simulink model "CAN_Model_v8"  (R2018b)
settings: Solver=VariableStepAuto  StartTime=0.0  StopTime=SimTime  RelTol=1e-3
values from neighbouring files (symbols this model uses):
  ID = [1,1,1,1,1,0,0,1,1,1,1]    [CAN_ModelMat.m]    (also in CAN_ModelMatv2.m; stuff.m = [ID(1:i) 0 ID(i+1:end)])
  ID_Rx = [1,1,1,1,0,0,1,1,1,1,1]    [CAN_ModelMat.m]    (also in CAN_ModelMatv2.m)
  NodesID = [ 0,0,1,1,0,1,1,0,0,1,1 ... (first row only)    [CAN_ModelMat.m]    (also in CAN_ModelMatv2.m)
  RTS_Inc = round(SimTime / CLK / NumOfFrames)    [CAN_ModelMat.m]    (also in CAN_ModelMatv2.m)
  time = NodeTiming / CLK    (= 5000)    [CAN_ModelMat.m]    (also in CAN_ModelMatv2.m)
libraries: simulink_extras x1
(part 1 of 2)
settings Model: Creator=Emiliano  LastModifiedBy=MAX_1

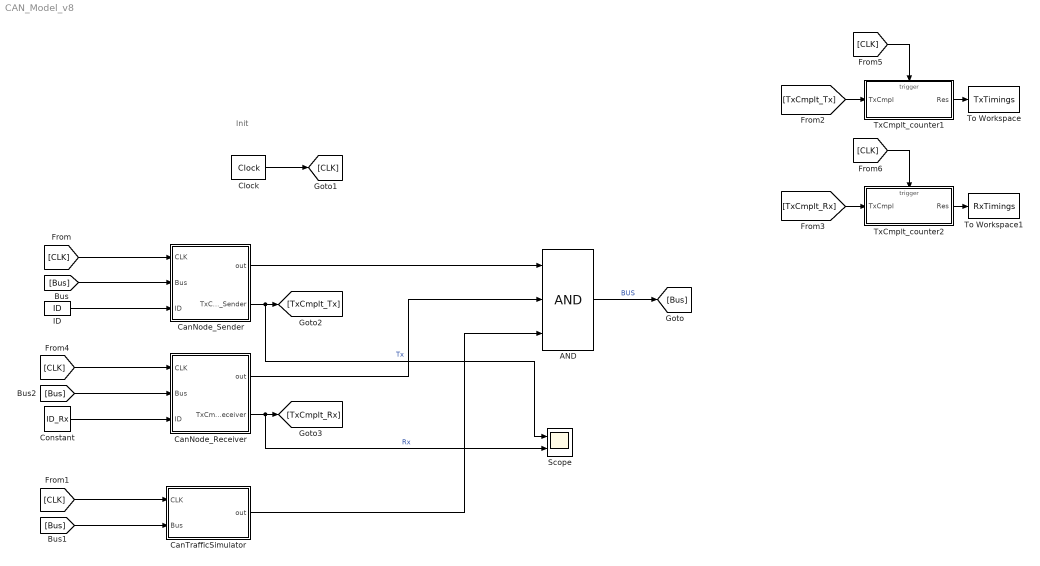
== system CAN_Model_v8 ==
  note: Init
  AND : Logic  Inputs=3  IconShape=distinctive  AllPortsSameDT=off  OutDataTypeStr=boolean
  CanNode_Receiver : Subsystem
  CanNode_Sender : Subsystem
  CanTrafficSimulator : Subsystem
  Clock : simulink_extras/Flip Flops/Clock  period=CLK
  Constant : Constant  Value=ID_Rx
  ID : Constant  Value=ID
  Scope : Scope  NumInputPorts=2
  To Workspace : ToWorkspace  VariableName=TxTimings  SaveFormat=Timeseries  SampleTime=-1
  To Workspace1 : ToWorkspace  VariableName=RxTimings  SaveFormat=Timeseries  SampleTime=-1
  TxCmplt_counter1 : Subsystem  TreatAsAtomicUnit=on
  TxCmplt_counter2 : Subsystem  TreatAsAtomicUnit=on
  wires:
  AND/1 -> [Bus]  "BUS"
  Clock/1 -> [CLK]
  [CLK] -> CanNode_Sender/1(CLK)
  [Bus] -> CanNode_Sender/2(Bus)
  ID/1 -> CanNode_Sender/3(ID)
  CanNode_Sender/1(out) -> AND/1
  [CLK] -> CanNode_Receiver/1(CLK)
  [Bus] -> CanNode_Receiver/2(Bus)
  Constant/1 -> CanNode_Receiver/3(ID)
  CanNode_Receiver/1(out) -> AND/2
  [CLK] -> CanTrafficSimulator/1(CLK)
  [Bus] -> CanTrafficSimulator/2("Bus ")
  CanTrafficSimulator/1(out) -> AND/3
  CanNode_Sender/2(TxCmplt_Sender) -> Scope/1, [TxCmplt_Tx]  "Tx"
  [CLK] -> TxCmplt_counter1/Trigger
  [CLK] -> TxCmplt_counter2/Trigger
  [TxCmplt_Rx] -> TxCmplt_counter2/1(TxCmpl)
  [TxCmplt_Tx] -> TxCmplt_counter1/1(TxCmpl)
  TxCmplt_counter1/1(Res) -> To Workspace/1
  TxCmplt_counter2/1(Res) -> To Workspace1/1
  CanNode_Receiver/2(TxCmplt_Receiver) -> Scope/2, [TxCmplt_Rx]  "Rx"

== system CAN_Model_v8/CanNode_Receiver ==
  CLK : Inport
  Bus : Inport  Port=2
  ID : Inport  Port=3
  CanNode : Subsystem
  Payload 1 : Constant  Value=[0,0,0,1,0,0,0,1,1,1,0,0,0,1,1,0,1,0,0,1,0,0,1,1,0,0,0,1,0,1,0,1,0,0,0,0,1,0,0,1,0,1,0,1,1,0,0,0,0,1,0,0,0,1,1,0,1,0,0,1,0,0,0,1]
  RTR2 : Constant
  Scope : Scope
  Triggered Subsystem2 : Subsystem  TreatAsAtomicUnit=on
  out : Outport
  TxCmplt_Receiver : Outport  Port=2
  wires:
  CanNode/3(txCmplt) -> TxCmplt_Receiver/1, Triggered Subsystem2/2(TxCmplt)  "TxCmplt_Receiver"
  Payload 1/1 -> CanNode/5(Data)
  RTR2/1 -> CanNode/4(RTR)
  CLK/1 -> Triggered Subsystem2/Trigger, CanNode/1(CLK)
  CanNode/2(DeStuffedFrame) -> Triggered Subsystem2/1(RxFrame)
  Triggered Subsystem2/1(RTS) -> Scope/1, CanNode/6("ReadyToSend ")  "RTS"
  CanNode/4(EOF) -> Triggered Subsystem2/3(EOF)
  ID/1 -> CanNode/3(ID)
  CanNode/1("TxBus ") -> out/1  "out"
  Bus/1 -> CanNode/2(Bus)

== system CAN_Model_v8/CanNode_Sender ==
  CLK : Inport
  Bus : Inport  Port=2
  ID : Inport  Port=3
  CanNode : Subsystem
  "Payload " : Constant  Value=[0,0,0,1,0,0,0,1,1,1,0,0,0,1,1,0,1,0,0,1,0,0,1,1,0,0,0,1,0,1,0,1,0,0,0,0,1,0,0,1,0,1,0,1,1,0,0,0,0,1,0,0,0,1,1,0,1,0,0,1,0,0,0,1]
  RTR : Constant
  RTS_Manager : Subsystem  TreatAsAtomicUnit=on
  Terminator : Terminator
  out : Outport
  TxCmplt_Sender : Outport  Port=2
  wires:
  Bus/1 -> CanNode/2(Bus)
  CLK/1 -> CanNode/1(CLK), RTS_Manager/Trigger
  "Payload "/1 -> CanNode/5(Data)
  CanNode/2(DeStuffedFrame) -> Terminator/1
  CanNode/1("TxBus ") -> out/1  "out"
  ID/1 -> CanNode/3(ID)
  CanNode/3(txCmplt) -> TxCmplt_Sender/1, RTS_Manager/1(TxCmplt)  "TxCmplt_Sender"
  RTS_Manager/1(RTS) -> CanNode/6("ReadyToSend ")  "RTS"
  RTR/1 -> CanNode/4(RTR)

== system CAN_Model_v8/CanTrafficSimulator ==
  CLK : Inport
  "Bus " : Inport  Port=2
  CanNode : Subsystem
  Payload 1 : Constant  Value=[0,0,0,1,0,0,0,1,1,1,0,0,0,1,1,0,1,0,0,1,0,0,1,1,0,0,0,1,0,1,0,1,0,0,0,0,1,0,0,1,0,1,0,1,1,0,0,0,0,1,0,0,0,1,1,0,1,0,0,1,0,0,0,1]
  RTR1 : Constant
  Terminator : Terminator
  To Workspace : ToWorkspace  VariableName=DeStuffed  SaveFormat=Timeseries  SampleTime=-1
  Triggered Subsystem : Subsystem  TreatAsAtomicUnit=on
  out : Outport
  wires:
  RTR1/1 -> CanNode/4(RTR)
  CanNode/2(DeStuffedFrame) -> To Workspace/1
  Triggered Subsystem/1(ID) -> CanNode/3(ID)
  CanNode/1("TxBus ") -> out/1  "out"
  CLK/1 -> CanNode/1(CLK), Triggered Subsystem/Trigger
  CanNode/3(txCmplt) -> Triggered Subsystem/1(TxCmplt)  "TxCmplt"
  "Bus "/1 -> CanNode/2(Bus)
  Triggered Subsystem/3(RTS) -> CanNode/6("ReadyToSend ")  "RTS_Traffic"
  Payload 1/1 -> CanNode/5(Data)
  Triggered Subsystem/2(RandPayload) -> Terminator/1

== system CAN_Model_v8/TxCmplt_counter1 ==
  TxCmpl : Inport
  Trigger : TriggerPort  VariantControl=Variant
  MATLAB Function : MATLAB Function  TreatAsAtomicUnit=on
  Memory : Memory  InitialCondition=1  InheritSampleTime=on
  Memory1 : Memory  InheritSampleTime=on
  Memory2 : Memory  InitialCondition=[0,0,0,0,0,0,0,0,0,0,0,0,0,0,0,0,0,0,0,0]  InheritSampleTime=on
  Res : Outport
  wires:
  MATLAB Function/3(nextIndex) -> Memory/1
  MATLAB Function/2(nextCount) -> Memory1/1
  MATLAB Function/1(nextRes) -> Res/1, Memory2/1
  Memory/1 -> MATLAB Function/4(index)
  Memory1/1 -> MATLAB Function/3(count)
  Memory2/1 -> MATLAB Function/2(Res)
  TxCmpl/1 -> MATLAB Function/1(TxCmplt)

== system CAN_Model_v8/TxCmplt_counter2 ==
  TxCmpl : Inport
  Trigger : TriggerPort  VariantControl=Variant
  MATLAB Function : MATLAB Function  TreatAsAtomicUnit=on
  Memory : Memory  InitialCondition=1  InheritSampleTime=on
  Memory1 : Memory  InheritSampleTime=on
  Memory2 : Memory  InitialCondition=[0,0,0,0,0,0,0,0,0,0,0,0,0,0,0,0,0,0,0,0]  InheritSampleTime=on
  Res : Outport
  wires:
  MATLAB Function/3(nextIndex) -> Memory/1
  MATLAB Function/2(nextCount) -> Memory1/1
  MATLAB Function/1(nextRes) -> Res/1, Memory2/1
  Memory/1 -> MATLAB Function/4(index)
  Memory1/1 -> MATLAB Function/3(count)
  Memory2/1 -> MATLAB Function/2(Res)
  TxCmpl/1 -> MATLAB Function/1(TxCmplt)

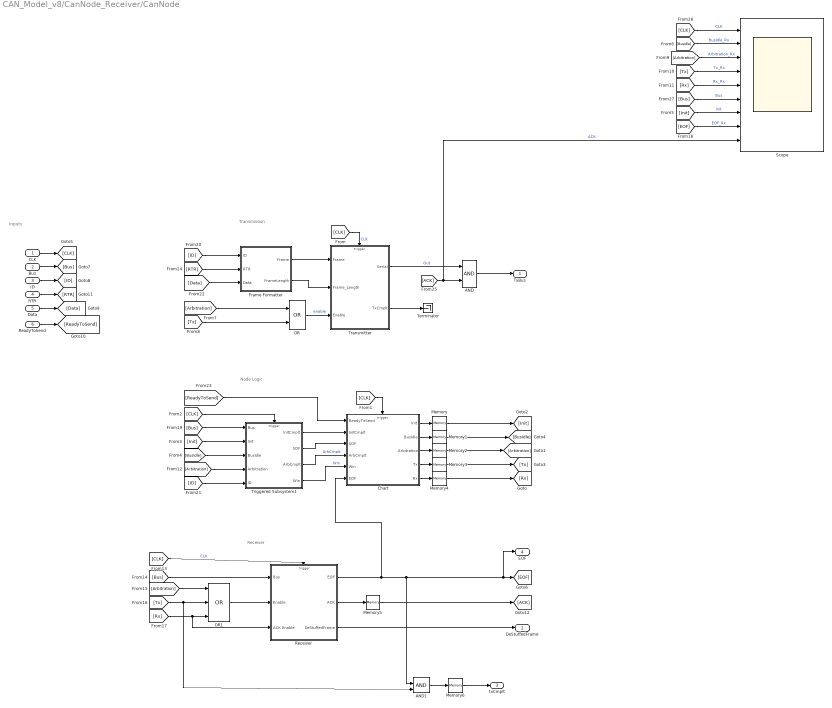
== system CAN_Model_v8/CanNode_Receiver/CanNode ==
  note: Transmission
  note: Node Logic
  note: Receiver
  note: Inputs
  CLK : Inport
  Bus : Inport  Port=2
  ID : Inport  Port=3
  RTR : Inport  Port=4
  Data : Inport  Port=5
  "ReadyToSend " : Inport  Port=6
  AND : Logic  IconShape=distinctive  AllPortsSameDT=off  OutDataTypeStr=boolean
  AND1 : Logic  IconShape=distinctive  AllPortsSameDT=off  OutDataTypeStr=boolean
  Chart : Stateflow chart  TreatAsAtomicUnit=on
  Frame Formatter : Subsystem
  Memory{,1..5} (6 alike) : Memory
  Memory6 : Memory  InheritSampleTime=on
  OR : Logic  Operator=OR  IconShape=distinctive  AllPortsSameDT=off  OutDataTypeStr=boolean
  OR1 : Logic  Operator=OR  Inputs=3  IconShape=distinctive  AllPortsSameDT=off  OutDataTypeStr=boolean
  Receiver : Subsystem  TreatAsAtomicUnit=on
  Scope : Scope  NumInputPorts=9
  Terminator : Terminator
  Transmitter : Subsystem  TreatAsAtomicUnit=on
  Triggered Subsystem1 : Subsystem  TreatAsAtomicUnit=on
  "TxBus " : Outport
  DeStuffedFrame : Outport  Port=2
  txCmplt : Outport  Port=3
  EOF : Outport  Port=4
  wires:
  [CLK] -> Chart/Trigger
  [Arbitration] -> OR/1
  [Tx] -> OR/2
  OR/1 -> Transmitter/3(Enable)  "enable"
  Chart/5(" Rx") -> Memory4/1
  Chart/3(" Arbitration") -> Memory2/1
  Chart/1(" Init") -> Memory/1
  Chart/4(" Tx") -> Memory3/1
  Chart/2(" BusIdle") -> Memory1/1
  CLK/1 -> [CLK]
  [CLK] -> Transmitter/Trigger  "CLK"
  [CLK] -> Triggered Subsystem1/Trigger
  [Init] -> Triggered Subsystem1/2(Init)
  [BusIdle] -> Triggered Subsystem1/3(BusIdle)
  Triggered Subsystem1/2(SOF) -> Chart/3(SOF)
  Triggered Subsystem1/3("ArbCmplt ") -> Chart/4(ArbCmplt)  "ArbCmplt"
  [CLK] -> Scope/1  "CLK"
  [BusIdle] -> Scope/2  "BusIdle_Rx"
  [Arbitration] -> Scope/3  "Arbitration_Rx"
  [Tx] -> Scope/4  "Tx_Rx"
  [Rx] -> Scope/5  "Rx_Rx"
  Memory/1 -> [Init]
  Memory1/1 -> [BusIdle]
  Memory2/1 -> [Arbitration]
  Memory3/1 -> [Tx]
  Memory4/1 -> [Rx]
  Transmitter/1(Serial) -> AND/1  "Out"
  [Arbitration] -> Triggered Subsystem1/4(Arbitration)
  [CLK] -> Receiver/Trigger  "CLK"
  [Bus] -> Receiver/1(Bus)
  [Arbitration] -> OR1/1
  [Tx] -> AND1/2, OR1/2
  Receiver/1(EOF) -> Chart/6(EOF), AND1/1, EOF/1, [EOF]
  [EOF] -> Scope/8  "EOF_Rx"
  Bus/1 -> [Bus]
  [Bus] -> Triggered Subsystem1/1(Bus)
  Frame Formatter/1(Frame) -> Transmitter/1("Frame ")
  Frame Formatter/2("FrameLength ") -> Transmitter/2(Frame_Length)
  ID/1 -> [ID]
  [ID] -> Frame Formatter/1(ID)
  [ID] -> Triggered Subsystem1/5(ID)
  Data/1 -> [Data]
  "ReadyToSend "/1 -> [ReadyToSend]
  [ReadyToSend] -> Chart/1(ReadyToSend)
  [Data] -> Frame Formatter/3(Data)
  RTR/1 -> [RTR]
  [RTR] -> Frame Formatter/2(RTR)
  Receiver/2(ACK) -> Memory5/1
  Triggered Subsystem1/4(Win) -> Chart/5(Win)  "Win"
  Memory5/1 -> [ACK]
  AND/1 -> "TxBus "/1
  [ACK] -> Scope/9, AND/2  "ACK"
  Triggered Subsystem1/1(InitCmplt) -> Chart/2(InitCmplt)
  [Init] -> Scope/7  "Init"
  Receiver/3(DeStuffedFrame) -> DeStuffedFrame/1
  OR1/1 -> Receiver/2(Enable)
  [Rx] -> Receiver/3(ACK Enable), OR1/3
  Transmitter/2(TxCmplt) -> Terminator/1
  AND1/1 -> Memory6/1
  Memory6/1 -> txCmplt/1
  [Bus] -> Scope/6  "Bus"

== system CAN_Model_v8/CanNode_Receiver/Triggered Subsystem2 ==
  RxFrame : Inport
  TxCmplt : Inport  Port=2
  EOF : Inport  Port=3
  Trigger : TriggerPort  VariantControl=Variant
  Constant : Constant  Value=ID
  MATLAB Function : MATLAB Function  TreatAsAtomicUnit=on
  Memory1 : Memory  InheritSampleTime=on
  Scope : Scope
  RTS : Outport
  wires:
  MATLAB Function/1(nextRTS) -> Memory1/1, RTS/1
  TxCmplt/1 -> MATLAB Function/2(TxCmplt)
  Memory1/1 -> MATLAB Function/5(RTS)
  EOF/1 -> MATLAB Function/3(EOF)
  RxFrame/1 -> MATLAB Function/4(RxFrame)
  Constant/1 -> MATLAB Function/1(MasterID)
  MATLAB Function/2(out) -> Scope/1

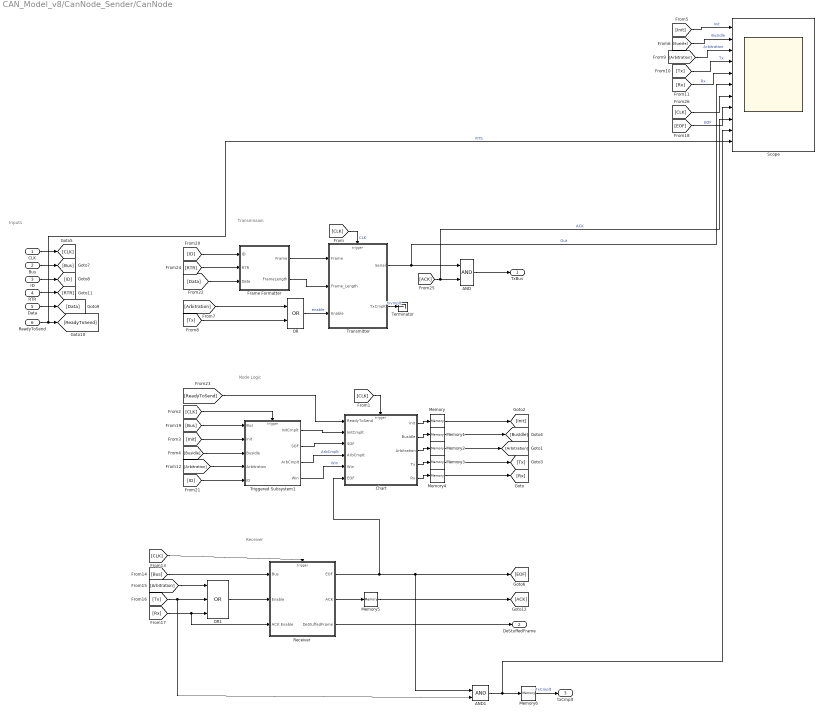
== system CAN_Model_v8/CanNode_Sender/CanNode ==
  note: Transmission
  note: Node Logic
  note: Receiver
  note: Inputs
  CLK : Inport
  Bus : Inport  Port=2
  ID : Inport  Port=3
  RTR : Inport  Port=4
  Data : Inport  Port=5
  "ReadyToSend " : Inport  Port=6
  AND : Logic  IconShape=distinctive  AllPortsSameDT=off  OutDataTypeStr=boolean
  AND1 : Logic  IconShape=distinctive  AllPortsSameDT=off  OutDataTypeStr=boolean
  Chart : Stateflow chart  TreatAsAtomicUnit=on
  Frame Formatter : Subsystem
  Memory{,1..5} (6 alike) : Memory
  Memory6 : Memory  InheritSampleTime=on
  OR : Logic  Operator=OR  IconShape=distinctive  AllPortsSameDT=off  OutDataTypeStr=boolean
  OR1 : Logic  Operator=OR  Inputs=3  IconShape=distinctive  AllPortsSameDT=off  OutDataTypeStr=boolean
  Receiver : Subsystem  TreatAsAtomicUnit=on
  Scope : Scope  NumInputPorts=11
  Terminator : Terminator
  Transmitter : Subsystem  TreatAsAtomicUnit=on
  Triggered Subsystem1 : Subsystem  TreatAsAtomicUnit=on
  "TxBus " : Outport
  DeStuffedFrame : Outport  Port=2
  txCmplt : Outport  Port=3
  wires:
  [CLK] -> Chart/Trigger
  [Arbitration] -> OR/1
  [Tx] -> OR/2
  OR/1 -> Transmitter/3(Enable)  "enable"
  Chart/5(" Rx") -> Memory4/1
  Chart/3(" Arbitration") -> Memory2/1
  Chart/1(" Init") -> Memory/1
  Chart/4(" Tx") -> Memory3/1
  Chart/2(" BusIdle") -> Memory1/1
  CLK/1 -> [CLK]
  [CLK] -> Transmitter/Trigger  "CLK"
  [CLK] -> Triggered Subsystem1/Trigger
  [Init] -> Triggered Subsystem1/2(Init)
  [BusIdle] -> Triggered Subsystem1/3(BusIdle)
  Triggered Subsystem1/2(SOF) -> Chart/3(SOF)
  Triggered Subsystem1/3("ArbCmplt ") -> Chart/4(ArbCmplt)  "ArbCmplt"
  [Init] -> Scope/1  "Init"
  [BusIdle] -> Scope/2  "BusIdle"
  [Arbitration] -> Scope/3  "Arbitration"
  [Tx] -> Scope/4  "Tx"
  [Rx] -> Scope/5  "Rx"
  Memory/1 -> [Init]
  Memory1/1 -> [BusIdle]
  Memory2/1 -> [Arbitration]
  Memory3/1 -> [Tx]
  Memory4/1 -> [Rx]
  Transmitter/1(Serial) -> Scope/6, AND/1  "Out"
  [Arbitration] -> Triggered Subsystem1/4(Arbitration)
  [CLK] -> Receiver/Trigger
  [Bus] -> Receiver/1(Bus)
  [Arbitration] -> OR1/1
  [Tx] -> AND1/2, OR1/2
  Receiver/1(EOF) -> Chart/6(EOF), AND1/1, [EOF]
  [EOF] -> Scope/8  "EOF"
  Bus/1 -> [Bus]
  [Bus] -> Triggered Subsystem1/1(Bus)
  Frame Formatter/1(Frame) -> Transmitter/1("Frame ")
  Frame Formatter/2("FrameLength ") -> Transmitter/2(Frame_Length)
  ID/1 -> [ID]
  [ID] -> Frame Formatter/1(ID)
  [ID] -> Triggered Subsystem1/5(ID)
  Data/1 -> [Data]
  "ReadyToSend "/1 -> Scope/11, [ReadyToSend]  "RTS"
  [ReadyToSend] -> Chart/1(ReadyToSend)
  [Data] -> Frame Formatter/3(Data)
  RTR/1 -> [RTR]
  [RTR] -> Frame Formatter/2(RTR)
  Receiver/2(ACK) -> Memory5/1
  Triggered Subsystem1/4(Win) -> Chart/5(Win)  "Win"
  Memory5/1 -> [ACK]
  AND/1 -> "TxBus "/1
  [ACK] -> Scope/9, AND/2  "ACK"
  Triggered Subsystem1/1(InitCmplt) -> Chart/2(InitCmplt)
  [CLK] -> Scope/7
  Receiver/3(DeStuffedFrame) -> DeStuffedFrame/1
  OR1/1 -> Receiver/2(Enable)
  [Rx] -> Receiver/3(ACK Enable), OR1/3
  Transmitter/2(TxCmplt) -> Terminator/1  "txvmplt"
  AND1/1 -> Scope/10, Memory6/1
  Memory6/1 -> txCmplt/1  "TxCmplt"

== system CAN_Model_v8/CanNode_Sender/RTS_Manager ==
  TxCmplt : Inport
  Trigger : TriggerPort  VariantControl=Variant
  Constant : Constant  Value=time
  MATLAB Function : MATLAB Function  TreatAsAtomicUnit=on
  Memory : Memory  InheritSampleTime=on
  Memory1 : Memory  InheritSampleTime=on
  Memory2 : Memory  InheritSampleTime=on
  RTS : Outport
  wires:
  MATLAB Function/1(nextRTS) -> Memory1/1, RTS/1
  Constant/1 -> MATLAB Function/1(Timer)
  TxCmplt/1 -> MATLAB Function/2(TxCmplt)
  MATLAB Function/2(nextCount) -> Memory/1
  Memory/1 -> MATLAB Function/4(Count)
  Memory1/1 -> MATLAB Function/3(RTS)
  MATLAB Function/3(nextNumPackets) -> Memory2/1
  Memory2/1 -> MATLAB Function/5(numPackets)

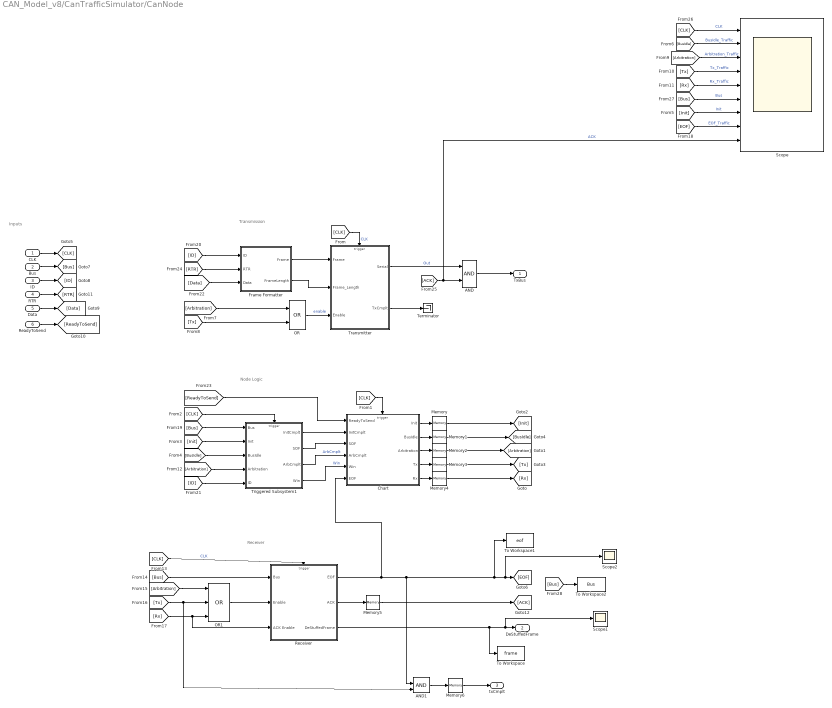
== system CAN_Model_v8/CanTrafficSimulator/CanNode ==
  note: Transmission
  note: Node Logic
  note: Receiver
  note: Inputs
  CLK : Inport
  Bus : Inport  Port=2
  ID : Inport  Port=3
  RTR : Inport  Port=4
  Data : Inport  Port=5
  "ReadyToSend " : Inport  Port=6
  AND : Logic  IconShape=distinctive  AllPortsSameDT=off  OutDataTypeStr=boolean
  AND1 : Logic  IconShape=distinctive  AllPortsSameDT=off  OutDataTypeStr=boolean
  Chart : Stateflow chart  TreatAsAtomicUnit=on
  Frame Formatter : Subsystem
  Memory{,1..5} (6 alike) : Memory
  Memory6 : Memory  InheritSampleTime=on
  OR : Logic  Operator=OR  IconShape=distinctive  AllPortsSameDT=off  OutDataTypeStr=boolean
  OR1 : Logic  Operator=OR  Inputs=3  IconShape=distinctive  AllPortsSameDT=off  OutDataTypeStr=boolean
  Receiver : Subsystem  TreatAsAtomicUnit=on
  Scope : Scope  NumInputPorts=9
  Scope1 : Scope
  Scope2 : Scope
  Terminator : Terminator
  To Workspace : ToWorkspace  VariableName=frame  SaveFormat=Timeseries  SampleTime=-1
  To Workspace1 : ToWorkspace  VariableName=eof  SaveFormat=Timeseries  SampleTime=-1
  To Workspace2 : ToWorkspace  VariableName=Bus  SaveFormat=Timeseries  SampleTime=-1
  Transmitter : Subsystem  TreatAsAtomicUnit=on
  Triggered Subsystem1 : Subsystem  TreatAsAtomicUnit=on
  "TxBus " : Outport
  DeStuffedFrame : Outport  Port=2
  txCmplt : Outport  Port=3
  wires:
  [CLK] -> Chart/Trigger
  [Arbitration] -> OR/1
  [Tx] -> OR/2
  OR/1 -> Transmitter/3(Enable)  "enable"
  Chart/5(" Rx") -> Memory4/1
  Chart/3(" Arbitration") -> Memory2/1
  Chart/1(" Init") -> Memory/1
  Chart/4(" Tx") -> Memory3/1
  Chart/2(" BusIdle") -> Memory1/1
  CLK/1 -> [CLK]
  [CLK] -> Transmitter/Trigger  "CLK"
  [CLK] -> Triggered Subsystem1/Trigger
  [Init] -> Triggered Subsystem1/2(Init)
  [BusIdle] -> Triggered Subsystem1/3(BusIdle)
  Triggered Subsystem1/2(SOF) -> Chart/3(SOF)
  Triggered Subsystem1/3("ArbCmplt ") -> Chart/4(ArbCmplt)  "ArbCmplt"
  [CLK] -> Scope/1  "CLK"
  [BusIdle] -> Scope/2  "BusIdle_Traffic"
  [Arbitration] -> Scope/3  "Arbitration_Traffic"
  [Tx] -> Scope/4  "Tx_Traffic"
  [Rx] -> Scope/5  "Rx_Traffic"
  Memory/1 -> [Init]
  Memory1/1 -> [BusIdle]
  Memory2/1 -> [Arbitration]
  Memory3/1 -> [Tx]
  Memory4/1 -> [Rx]
  Transmitter/1(Serial) -> AND/1  "Out"
  [Arbitration] -> Triggered Subsystem1/4(Arbitration)
  [CLK] -> Receiver/Trigger  "CLK"
  [Bus] -> Receiver/1(Bus)
  [Arbitration] -> OR1/1
  [Tx] -> AND1/2, OR1/2
  Receiver/1(EOF) -> Chart/6(EOF), AND1/1, To Workspace1/1, Scope2/1, [EOF]
  [EOF] -> Scope/8  "EOF_Traffic"
  Bus/1 -> [Bus]
  [Bus] -> Triggered Subsystem1/1(Bus)
  Frame Formatter/1(Frame) -> Transmitter/1("Frame ")
  Frame Formatter/2("FrameLength ") -> Transmitter/2(Frame_Length)
  ID/1 -> [ID]
  [ID] -> Frame Formatter/1(ID)
  [ID] -> Triggered Subsystem1/5(ID)
  Data/1 -> [Data]
  "ReadyToSend "/1 -> [ReadyToSend]
  [ReadyToSend] -> Chart/1(ReadyToSend)
  [Data] -> Frame Formatter/3(Data)
  RTR/1 -> [RTR]
  [RTR] -> Frame Formatter/2(RTR)
  Receiver/2(ACK) -> Memory5/1
  Triggered Subsystem1/4(Win) -> Chart/5(Win)  "Win"
  Memory5/1 -> [ACK]
  AND/1 -> "TxBus "/1
  [ACK] -> Scope/9, AND/2  "ACK"
  Triggered Subsystem1/1(InitCmplt) -> Chart/2(InitCmplt)
  [Init] -> Scope/7  "Init"
  Receiver/3(DeStuffedFrame) -> To Workspace/1, Scope1/1, DeStuffedFrame/1
  OR1/1 -> Receiver/2(Enable)
  [Rx] -> Receiver/3(ACK Enable), OR1/3
  Transmitter/2(TxCmplt) -> Terminator/1
  AND1/1 -> Memory6/1
  Memory6/1 -> txCmplt/1
  [Bus] -> Scope/6  "Bus"
  [Bus] -> To Workspace2/1

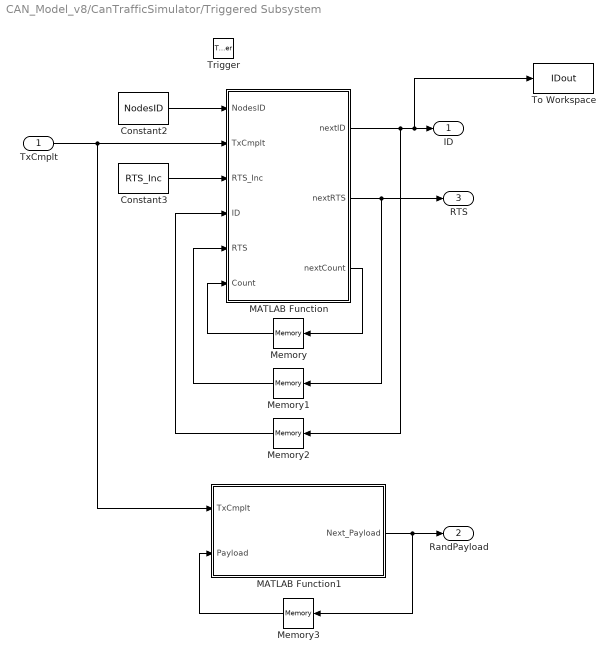
== system CAN_Model_v8/CanTrafficSimulator/Triggered Subsystem ==
  TxCmplt : Inport
  Trigger : TriggerPort  VariantControl=Variant
  Constant2 : Constant  Value=NodesID
  Constant3 : Constant  Value=RTS_Inc
  MATLAB Function : MATLAB Function  TreatAsAtomicUnit=on
  MATLAB Function1 : MATLAB Function  TreatAsAtomicUnit=on
  Memory : Memory  InheritSampleTime=on
  Memory1 : Memory  InheritSampleTime=on
  Memory2 : Memory  InitialCondition=NodesID(1,:)  InheritSampleTime=on
  Memory3 : Memory  InitialCondition=randi([0,1],64, 1)  InheritSampleTime=on
  To Workspace : ToWorkspace  VariableName=IDout  SaveFormat=Timeseries  SampleTime=-1
  ID : Outport
  RandPayload : Outport  Port=2
  RTS : Outport  Port=3
  wires:
  Constant2/1 -> MATLAB Function/1(NodesID)
  MATLAB Function/3(nextCount) -> Memory/1
  Memory/1 -> MATLAB Function/6(Count)
  MATLAB Function/2(nextRTS) -> Memory1/1, RTS/1
  Memory1/1 -> MATLAB Function/5(RTS)
  MATLAB Function/1(nextID) -> To Workspace/1, ID/1, Memory2/1
  Memory2/1 -> MATLAB Function/4(ID)
  Constant3/1 -> MATLAB Function/3(RTS_Inc)
  TxCmplt/1 -> MATLAB Function1/1(TxCmplt), MATLAB Function/2(TxCmplt)
  MATLAB Function1/1(Next_Payload) -> RandPayload/1, Memory3/1
  Memory3/1 -> MATLAB Function1/2(Payload)

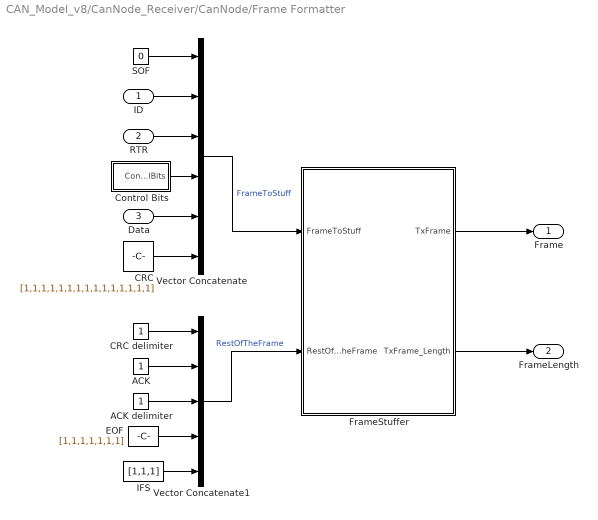
== system CAN_Model_v8/CanNode_Receiver/CanNode/Frame Formatter ==
  ID : Inport
  RTR : Inport  Port=2
  Data : Inport  Port=3
  ACK : Constant
  ACK delimiter : Constant
  CRC : Constant  Value=[1,1,1,1,1,1,1,1,1,1,1,1,1,1,1]
  CRC delimiter : Constant  VectorParams1D=off
  Control Bits : Subsystem
  EOF : Constant  Value=[1,1,1,1,1,1,1]
  FrameStuffer : Subsystem
  IFS : Constant  Value=[1,1,1]
  SOF : Constant  Value=0
  Vector Concatenate : Concatenate  NumInputs=6
  Vector Concatenate1 : Concatenate  NumInputs=5
  Frame : Outport
  "FrameLength " : Outport  Port=2
  wires:
  ID/1 -> Vector Concatenate/2
  RTR/1 -> Vector Concatenate/3
  Vector Concatenate/1 -> FrameStuffer/1(FrameToStuff)  "FrameToStuff"
  FrameStuffer/1(TxFrame) -> Frame/1
  FrameStuffer/2(TxFrame_Length) -> "FrameLength "/1
  SOF/1 -> Vector Concatenate/1
  Control Bits/1(ControlBits) -> Vector Concatenate/4
  Data/1 -> Vector Concatenate/5
  CRC/1 -> Vector Concatenate/6
  CRC delimiter/1 -> Vector Concatenate1/1
  ACK/1 -> Vector Concatenate1/2
  ACK delimiter/1 -> Vector Concatenate1/3
  EOF/1 -> Vector Concatenate1/4
  IFS/1 -> Vector Concatenate1/5
  Vector Concatenate1/1 -> FrameStuffer/2(RestOfTheFrame)  "RestOfTheFrame"

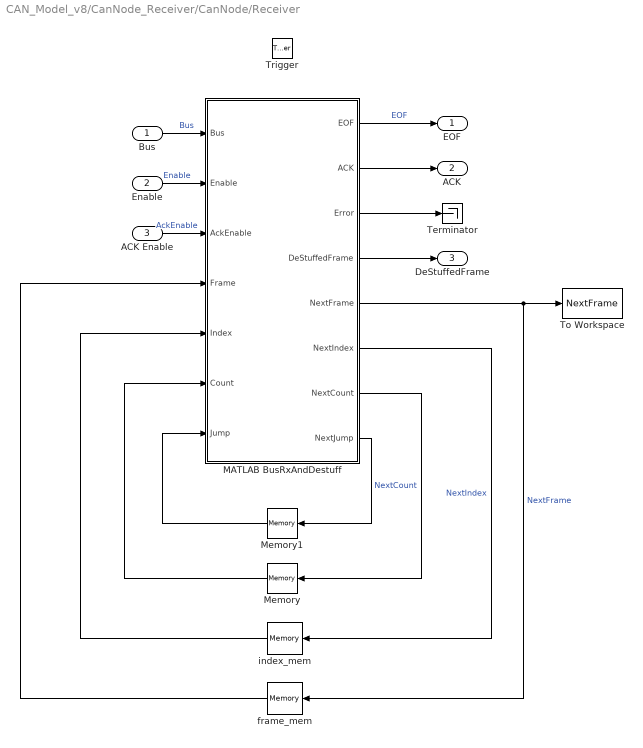
== system CAN_Model_v8/CanNode_Receiver/CanNode/Receiver ==
  Bus : Inport
  Enable : Inport  Port=2
  ACK Enable : Inport  Port=3
  Trigger : TriggerPort  VariantControl=Variant
  MATLAB BusRxAndDestuff : MATLAB Function  TreatAsAtomicUnit=on
  Memory : Memory  InheritSampleTime=on
  Memory1 : Memory  InheritSampleTime=on
  Terminator : Terminator
  To Workspace : ToWorkspace  VariableName=NextFrame  SaveFormat=Timeseries  SampleTime=-1
  frame_mem : Memory  InitialCondition=[0,0,0,0,0,0,0,0,0,0,0,0,0,0,0,0,0,0,0,0,0,0,0,0,0,0,0,0,0,0,0,0,0,0,0,0,0,0,0,0,0,0,0,0,0,0,0,0,0,0,0,0,0,0,0,0,0,0,0,0,0,0,0,0,0,0,0,0,0,0,0,0,0,0,0,0,0,0,0,0,0,0,0,0,0,0,0,0,0,0,0,0,0,0,0,0,0,0,0,0,0,0,0,0,0,0,0,0,0,0,0]  InheritSampleTime=on
  index_mem : Memory  InitialCondition=2  InheritSampleTime=on
  EOF : Outport
  ACK : Outport  Port=2
  DeStuffedFrame : Outport  Port=3
  wires:
  Enable/1 -> MATLAB BusRxAndDestuff/2(Enable)  "Enable"
  Bus/1 -> MATLAB BusRxAndDestuff/1(Bus)  "Bus"
  MATLAB BusRxAndDestuff/6(NextIndex) -> index_mem/1  "NextIndex"
  frame_mem/1 -> MATLAB BusRxAndDestuff/4(Frame)
  MATLAB BusRxAndDestuff/1(EOF) -> EOF/1  "EOF"
  MATLAB BusRxAndDestuff/5(NextFrame) -> To Workspace/1, frame_mem/1  "NextFrame"
  index_mem/1 -> MATLAB BusRxAndDestuff/5(Index)
  MATLAB BusRxAndDestuff/3(Error) -> Terminator/1
  MATLAB BusRxAndDestuff/7(NextCount) -> Memory/1  "NextCount"
  Memory/1 -> MATLAB BusRxAndDestuff/6(Count)
  MATLAB BusRxAndDestuff/8(NextJump) -> Memory1/1
  Memory1/1 -> MATLAB BusRxAndDestuff/7(Jump)
  MATLAB BusRxAndDestuff/4(DeStuffedFrame) -> DeStuffedFrame/1
  MATLAB BusRxAndDestuff/2(ACK) -> ACK/1
  ACK Enable/1 -> MATLAB BusRxAndDestuff/3(AckEnable)  "AckEnable"

== system CAN_Model_v8/CanNode_Receiver/CanNode/Transmitter ==
  "Frame " : Inport
  Frame_Length : Inport  Port=2
  Enable : Inport  Port=3
  Trigger : TriggerPort  VariantControl=Variant
  CAN_Transmission : MATLAB Function  TreatAsAtomicUnit=on
  Memory1 : Memory  InitialCondition=1  InheritSampleTime=on
  Serial : Outport
  TxCmplt : Outport  Port=2
  wires:
  Memory1/1 -> CAN_Transmission/4(index)
  CAN_Transmission/1(serial) -> Serial/1
  CAN_Transmission/3(next_index) -> Memory1/1
  CAN_Transmission/2(tx_completed) -> TxCmplt/1
  Enable/1 -> CAN_Transmission/3(enable)
  "Frame "/1 -> CAN_Transmission/1(frame)
  Frame_Length/1 -> CAN_Transmission/2(frame_length)

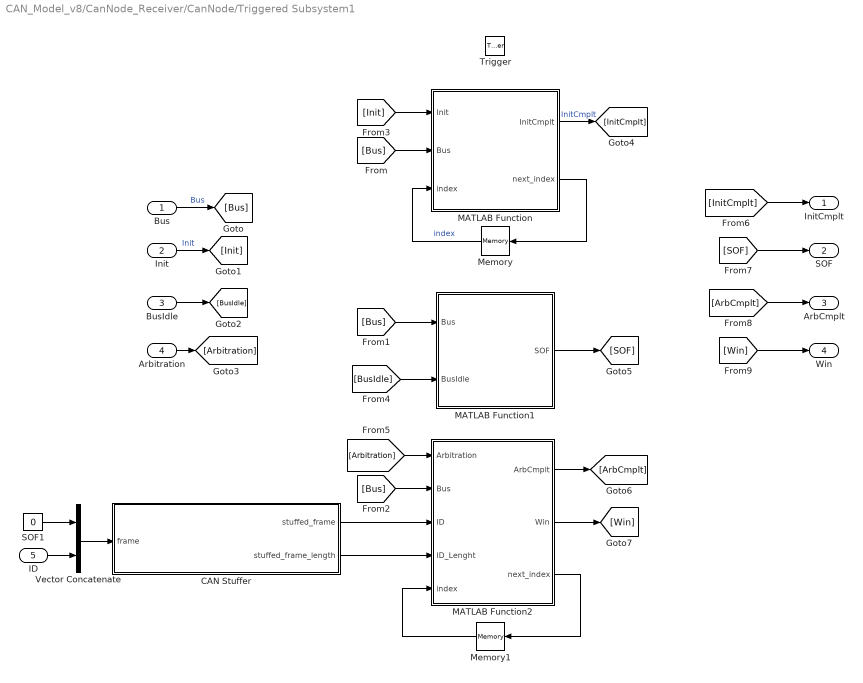
== system CAN_Model_v8/CanNode_Receiver/CanNode/Triggered Subsystem1 ==
  Bus : Inport
  Init : Inport  Port=2
  BusIdle : Inport  Port=3
  Arbitration : Inport  Port=4
  ID : Inport  Port=5
  Trigger : TriggerPort  VariantControl=Variant
  CAN Stuffer : MATLAB Function  TreatAsAtomicUnit=on
  MATLAB Function : MATLAB Function  TreatAsAtomicUnit=on
  MATLAB Function1 : MATLAB Function  TreatAsAtomicUnit=on
  MATLAB Function2 : MATLAB Function  TreatAsAtomicUnit=on
  Memory : Memory  InheritSampleTime=on
  Memory1 : Memory  InitialCondition=1  InheritSampleTime=on
  SOF1 : Constant  Value=0
  Vector Concatenate : Concatenate
  InitCmplt : Outport
  SOF : Outport  Port=2
  "ArbCmplt " : Outport  Port=3
  Win : Outport  Port=4
  wires:
  MATLAB Function/2(next_index) -> Memory/1
  Memory/1 -> MATLAB Function/3(index)  "index"
  Bus/1 -> [Bus]  "Bus"
  [Bus] -> MATLAB Function/2(Bus)
  [Bus] -> MATLAB Function1/1(Bus)
  [Bus] -> MATLAB Function2/2(Bus)
  MATLAB Function2/3(next_index) -> Memory1/1
  Memory1/1 -> MATLAB Function2/5(index)
  CAN Stuffer/1(stuffed_frame) -> MATLAB Function2/3(ID)
  CAN Stuffer/2(stuffed_frame_length) -> MATLAB Function2/4(ID_Lenght)
  SOF1/1 -> Vector Concatenate/1
  ID/1 -> Vector Concatenate/2
  Vector Concatenate/1 -> CAN Stuffer/1(frame)
  Init/1 -> [Init]  "Init"
  [Init] -> MATLAB Function/1(Init)
  BusIdle/1 -> [BusIdle]
  [BusIdle] -> MATLAB Function1/2(BusIdle)
  Arbitration/1 -> [Arbitration]
  [Arbitration] -> MATLAB Function2/1(Arbitration)
  MATLAB Function/1(InitCmplt) -> [InitCmplt]  "InitCmplt"
  [InitCmplt] -> InitCmplt/1
  MATLAB Function1/1(SOF) -> [SOF]
  [SOF] -> SOF/1
  MATLAB Function2/1(ArbCmplt) -> [ArbCmplt]
  [ArbCmplt] -> "ArbCmplt "/1
  [Win] -> Win/1
  MATLAB Function2/2(Win) -> [Win]

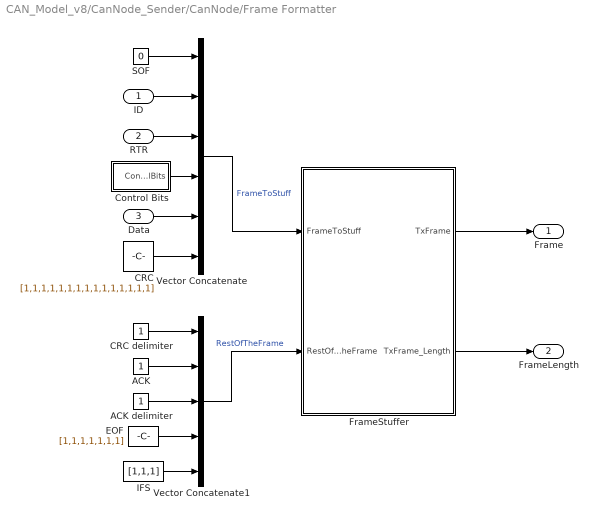
== system CAN_Model_v8/CanNode_Sender/CanNode/Frame Formatter ==
  ID : Inport
  RTR : Inport  Port=2
  Data : Inport  Port=3
  ACK : Constant
  ACK delimiter : Constant
  CRC : Constant  Value=[1,1,1,1,1,1,1,1,1,1,1,1,1,1,1]
  CRC delimiter : Constant  VectorParams1D=off
  Control Bits : Subsystem
  EOF : Constant  Value=[1,1,1,1,1,1,1]
  FrameStuffer : Subsystem
  IFS : Constant  Value=[1,1,1]
  SOF : Constant  Value=0
  Vector Concatenate : Concatenate  NumInputs=6
  Vector Concatenate1 : Concatenate  NumInputs=5
  Frame : Outport
  "FrameLength " : Outport  Port=2
  wires:
  ID/1 -> Vector Concatenate/2
  RTR/1 -> Vector Concatenate/3
  Vector Concatenate/1 -> FrameStuffer/1(FrameToStuff)  "FrameToStuff"
  FrameStuffer/1(TxFrame) -> Frame/1
  FrameStuffer/2(TxFrame_Length) -> "FrameLength "/1
  SOF/1 -> Vector Concatenate/1
  Control Bits/1(ControlBits) -> Vector Concatenate/4
  Data/1 -> Vector Concatenate/5
  CRC/1 -> Vector Concatenate/6
  CRC delimiter/1 -> Vector Concatenate1/1
  ACK/1 -> Vector Concatenate1/2
  ACK delimiter/1 -> Vector Concatenate1/3
  EOF/1 -> Vector Concatenate1/4
  IFS/1 -> Vector Concatenate1/5
  Vector Concatenate1/1 -> FrameStuffer/2(RestOfTheFrame)  "RestOfTheFrame"

== system CAN_Model_v8/CanNode_Sender/CanNode/Receiver ==
  Bus : Inport
  Enable : Inport  Port=2
  ACK Enable : Inport  Port=3
  Trigger : TriggerPort  VariantControl=Variant
  MATLAB BusRxAndDestuff : MATLAB Function  TreatAsAtomicUnit=on
  Memory : Memory  InheritSampleTime=on
  Memory1 : Memory  InheritSampleTime=on
  Terminator : Terminator
  frame_mem : Memory  InitialCondition=[0,0,0,0,0,0,0,0,0,0,0,0,0,0,0,0,0,0,0,0,0,0,0,0,0,0,0,0,0,0,0,0,0,0,0,0,0,0,0,0,0,0,0,0,0,0,0,0,0,0,0,0,0,0,0,0,0,0,0,0,0,0,0,0,0,0,0,0,0,0,0,0,0,0,0,0,0,0,0,0,0,0,0,0,0,0,0,0,0,0,0,0,0,0,0,0,0,0,0,0,0,0,0,0,0,0,0,0,0,0,0]  InheritSampleTime=on
  index_mem : Memory  InitialCondition=2  InheritSampleTime=on
  EOF : Outport
  ACK : Outport  Port=2
  DeStuffedFrame : Outport  Port=3
  wires:
  Enable/1 -> MATLAB BusRxAndDestuff/2(Enable)
  Bus/1 -> MATLAB BusRxAndDestuff/1(Bus)
  MATLAB BusRxAndDestuff/6(NextIndex) -> index_mem/1
  frame_mem/1 -> MATLAB BusRxAndDestuff/4(Frame)
  MATLAB BusRxAndDestuff/1(EOF) -> EOF/1
  MATLAB BusRxAndDestuff/5(NextFrame) -> frame_mem/1
  index_mem/1 -> MATLAB BusRxAndDestuff/5(Index)
  MATLAB BusRxAndDestuff/3(Error) -> Terminator/1
  MATLAB BusRxAndDestuff/7(NextCount) -> Memory/1
  Memory/1 -> MATLAB BusRxAndDestuff/6(Count)
  MATLAB BusRxAndDestuff/8(NextJump) -> Memory1/1
  Memory1/1 -> MATLAB BusRxAndDestuff/7(Jump)
  MATLAB BusRxAndDestuff/4(DeStuffedFrame) -> DeStuffedFrame/1
  MATLAB BusRxAndDestuff/2(ACK) -> ACK/1
  ACK Enable/1 -> MATLAB BusRxAndDestuff/3(AckEnable)

== system CAN_Model_v8/CanNode_Sender/CanNode/Transmitter ==
  "Frame " : Inport
  Frame_Length : Inport  Port=2
  Enable : Inport  Port=3
  Trigger : TriggerPort  VariantControl=Variant
  CAN_Transmission : MATLAB Function  TreatAsAtomicUnit=on
  Memory1 : Memory  InitialCondition=1  InheritSampleTime=on
  Serial : Outport
  TxCmplt : Outport  Port=2
  wires:
  Memory1/1 -> CAN_Transmission/4(index)
  CAN_Transmission/1(serial) -> Serial/1
  CAN_Transmission/3(next_index) -> Memory1/1
  CAN_Transmission/2(tx_completed) -> TxCmplt/1
  Enable/1 -> CAN_Transmission/3(enable)
  "Frame "/1 -> CAN_Transmission/1(frame)
  Frame_Length/1 -> CAN_Transmission/2(frame_length)

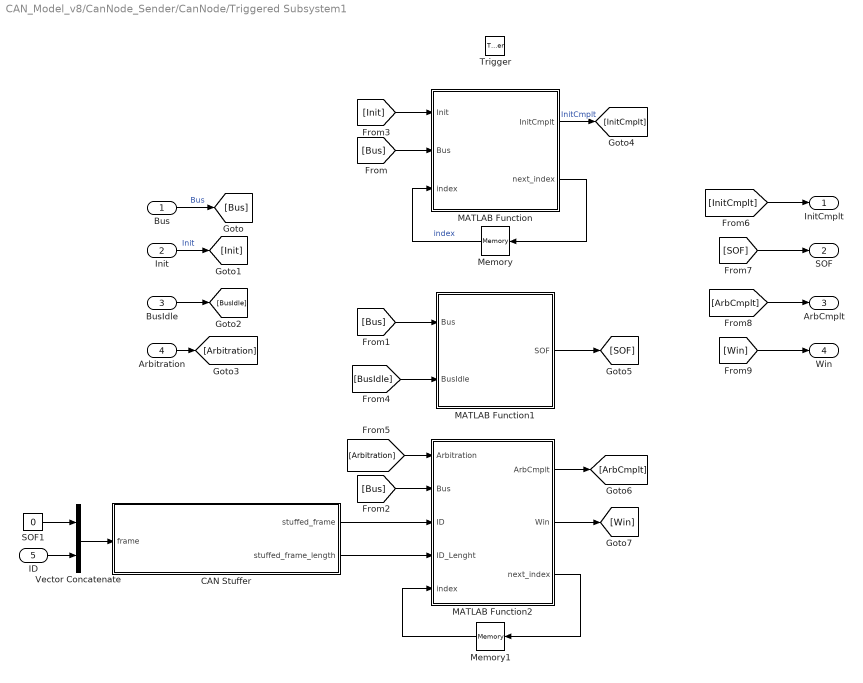
== system CAN_Model_v8/CanNode_Sender/CanNode/Triggered Subsystem1 ==
  Bus : Inport
  Init : Inport  Port=2
  BusIdle : Inport  Port=3
  Arbitration : Inport  Port=4
  ID : Inport  Port=5
  Trigger : TriggerPort  VariantControl=Variant
  CAN Stuffer : MATLAB Function  TreatAsAtomicUnit=on
  MATLAB Function : MATLAB Function  TreatAsAtomicUnit=on
  MATLAB Function1 : MATLAB Function  TreatAsAtomicUnit=on
  MATLAB Function2 : MATLAB Function  TreatAsAtomicUnit=on
  Memory : Memory  InheritSampleTime=on
  Memory1 : Memory  InitialCondition=1  InheritSampleTime=on
  SOF1 : Constant  Value=0
  Vector Concatenate : Concatenate
  InitCmplt : Outport
  SOF : Outport  Port=2
  "ArbCmplt " : Outport  Port=3
  Win : Outport  Port=4
  wires:
  MATLAB Function/2(next_index) -> Memory/1
  Memory/1 -> MATLAB Function/3(index)  "index"
  Bus/1 -> [Bus]  "Bus"
  [Bus] -> MATLAB Function/2(Bus)
  [Bus] -> MATLAB Function1/1(Bus)
  [Bus] -> MATLAB Function2/2(Bus)
  MATLAB Function2/3(next_index) -> Memory1/1
  Memory1/1 -> MATLAB Function2/5(index)
  CAN Stuffer/1(stuffed_frame) -> MATLAB Function2/3(ID)
  CAN Stuffer/2(stuffed_frame_length) -> MATLAB Function2/4(ID_Lenght)
  SOF1/1 -> Vector Concatenate/1
  ID/1 -> Vector Concatenate/2
  Vector Concatenate/1 -> CAN Stuffer/1(frame)
  Init/1 -> [Init]  "Init"
  [Init] -> MATLAB Function/1(Init)
  BusIdle/1 -> [BusIdle]
  [BusIdle] -> MATLAB Function1/2(BusIdle)
  Arbitration/1 -> [Arbitration]
  [Arbitration] -> MATLAB Function2/1(Arbitration)
  MATLAB Function/1(InitCmplt) -> [InitCmplt]  "InitCmplt"
  [InitCmplt] -> InitCmplt/1
  MATLAB Function1/1(SOF) -> [SOF]
  [SOF] -> SOF/1
  MATLAB Function2/1(ArbCmplt) -> [ArbCmplt]
  [ArbCmplt] -> "ArbCmplt "/1
  [Win] -> Win/1
  MATLAB Function2/2(Win) -> [Win]

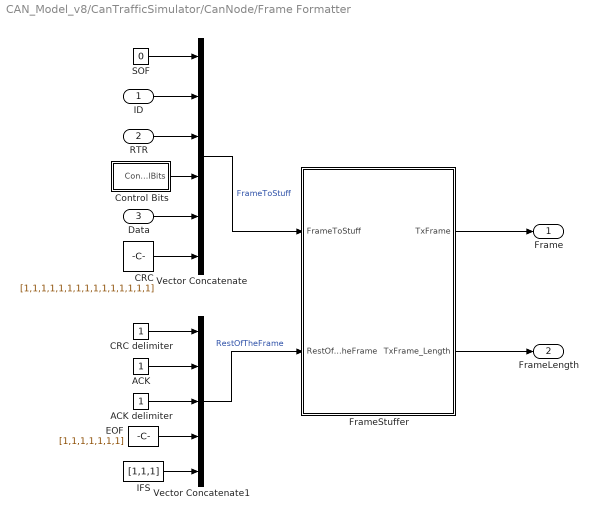
== system CAN_Model_v8/CanTrafficSimulator/CanNode/Frame Formatter ==
  ID : Inport
  RTR : Inport  Port=2
  Data : Inport  Port=3
  ACK : Constant
  ACK delimiter : Constant
  CRC : Constant  Value=[1,1,1,1,1,1,1,1,1,1,1,1,1,1,1]
  CRC delimiter : Constant  VectorParams1D=off
  Control Bits : Subsystem
  EOF : Constant  Value=[1,1,1,1,1,1,1]
  FrameStuffer : Subsystem
  IFS : Constant  Value=[1,1,1]
  SOF : Constant  Value=0
  Vector Concatenate : Concatenate  NumInputs=6
  Vector Concatenate1 : Concatenate  NumInputs=5
  Frame : Outport
  "FrameLength " : Outport  Port=2
  wires:
  ID/1 -> Vector Concatenate/2
  RTR/1 -> Vector Concatenate/3
  Vector Concatenate/1 -> FrameStuffer/1(FrameToStuff)  "FrameToStuff"
  FrameStuffer/1(TxFrame) -> Frame/1
  FrameStuffer/2(TxFrame_Length) -> "FrameLength "/1
  SOF/1 -> Vector Concatenate/1
  Control Bits/1(ControlBits) -> Vector Concatenate/4
  Data/1 -> Vector Concatenate/5
  CRC/1 -> Vector Concatenate/6
  CRC delimiter/1 -> Vector Concatenate1/1
  ACK/1 -> Vector Concatenate1/2
  ACK delimiter/1 -> Vector Concatenate1/3
  EOF/1 -> Vector Concatenate1/4
  IFS/1 -> Vector Concatenate1/5
  Vector Concatenate1/1 -> FrameStuffer/2(RestOfTheFrame)  "RestOfTheFrame"

== system CAN_Model_v8/CanTrafficSimulator/CanNode/Receiver ==
  Bus : Inport
  Enable : Inport  Port=2
  ACK Enable : Inport  Port=3
  Trigger : TriggerPort  VariantControl=Variant
  MATLAB BusRxAndDestuff : MATLAB Function  TreatAsAtomicUnit=on
  Memory : Memory  InheritSampleTime=on
  Memory1 : Memory  InheritSampleTime=on
  Terminator : Terminator
  frame_mem : Memory  InitialCondition=[0,0,0,0,0,0,0,0,0,0,0,0,0,0,0,0,0,0,0,0,0,0,0,0,0,0,0,0,0,0,0,0,0,0,0,0,0,0,0,0,0,0,0,0,0,0,0,0,0,0,0,0,0,0,0,0,0,0,0,0,0,0,0,0,0,0,0,0,0,0,0,0,0,0,0,0,0,0,0,0,0,0,0,0,0,0,0,0,0,0,0,0,0,0,0,0,0,0,0,0,0,0,0,0,0,0,0,0,0,0,0]  InheritSampleTime=on
  index_mem : Memory  InitialCondition=2  InheritSampleTime=on
  EOF : Outport
  ACK : Outport  Port=2
  DeStuffedFrame : Outport  Port=3
  wires:
  Enable/1 -> MATLAB BusRxAndDestuff/2(Enable)  "Enable"
  Bus/1 -> MATLAB BusRxAndDestuff/1(Bus)  "Bus"
  MATLAB BusRxAndDestuff/6(NextIndex) -> index_mem/1  "NextIndex"
  frame_mem/1 -> MATLAB BusRxAndDestuff/4(Frame)
  MATLAB BusRxAndDestuff/1(EOF) -> EOF/1  "EOF"
  MATLAB BusRxAndDestuff/5(NextFrame) -> frame_mem/1  "NextFrame"
  index_mem/1 -> MATLAB BusRxAndDestuff/5(Index)
  MATLAB BusRxAndDestuff/3(Error) -> Terminator/1
  MATLAB BusRxAndDestuff/7(NextCount) -> Memory/1  "NextCount"
  Memory/1 -> MATLAB BusRxAndDestuff/6(Count)
  MATLAB BusRxAndDestuff/8(NextJump) -> Memory1/1
  Memory1/1 -> MATLAB BusRxAndDestuff/7(Jump)
  MATLAB BusRxAndDestuff/4(DeStuffedFrame) -> DeStuffedFrame/1
  MATLAB BusRxAndDestuff/2(ACK) -> ACK/1
  ACK Enable/1 -> MATLAB BusRxAndDestuff/3(AckEnable)  "AckEnable"

== system CAN_Model_v8/CanTrafficSimulator/CanNode/Transmitter ==
  "Frame " : Inport
  Frame_Length : Inport  Port=2
  Enable : Inport  Port=3
  Trigger : TriggerPort  VariantControl=Variant
  CAN_Transmission : MATLAB Function  TreatAsAtomicUnit=on
  Memory1 : Memory  InitialCondition=1  InheritSampleTime=on
  Serial : Outport
  TxCmplt : Outport  Port=2
  wires:
  Memory1/1 -> CAN_Transmission/4(index)
  CAN_Transmission/1(serial) -> Serial/1
  CAN_Transmission/3(next_index) -> Memory1/1
  CAN_Transmission/2(tx_completed) -> TxCmplt/1
  Enable/1 -> CAN_Transmission/3(enable)
  "Frame "/1 -> CAN_Transmission/1(frame)
  Frame_Length/1 -> CAN_Transmission/2(frame_length)

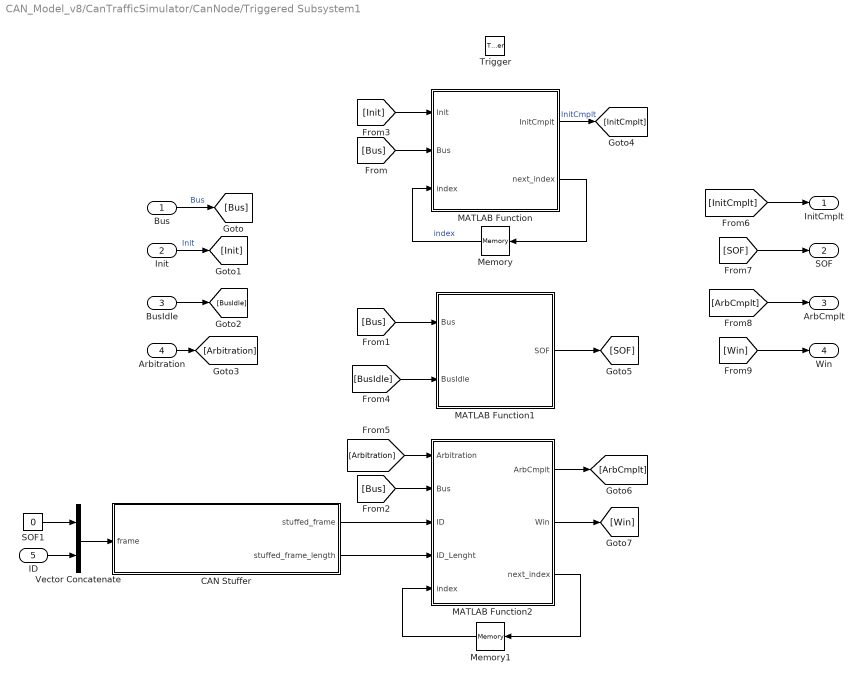
== system CAN_Model_v8/CanTrafficSimulator/CanNode/Triggered Subsystem1 ==
  Bus : Inport
  Init : Inport  Port=2
  BusIdle : Inport  Port=3
  Arbitration : Inport  Port=4
  ID : Inport  Port=5
  Trigger : TriggerPort  VariantControl=Variant
  CAN Stuffer : MATLAB Function  TreatAsAtomicUnit=on
  MATLAB Function : MATLAB Function  TreatAsAtomicUnit=on
  MATLAB Function1 : MATLAB Function  TreatAsAtomicUnit=on
  MATLAB Function2 : MATLAB Function  TreatAsAtomicUnit=on
  Memory : Memory  InheritSampleTime=on
  Memory1 : Memory  InitialCondition=1  InheritSampleTime=on
  SOF1 : Constant  Value=0
  Vector Concatenate : Concatenate
  InitCmplt : Outport
  SOF : Outport  Port=2
  "ArbCmplt " : Outport  Port=3
  Win : Outport  Port=4
  wires:
  MATLAB Function/2(next_index) -> Memory/1
  Memory/1 -> MATLAB Function/3(index)  "index"
  Bus/1 -> [Bus]  "Bus"
  [Bus] -> MATLAB Function/2(Bus)
  [Bus] -> MATLAB Function1/1(Bus)
  [Bus] -> MATLAB Function2/2(Bus)
  MATLAB Function2/3(next_index) -> Memory1/1
  Memory1/1 -> MATLAB Function2/5(index)
  CAN Stuffer/1(stuffed_frame) -> MATLAB Function2/3(ID)
  CAN Stuffer/2(stuffed_frame_length) -> MATLAB Function2/4(ID_Lenght)
  SOF1/1 -> Vector Concatenate/1
  ID/1 -> Vector Concatenate/2
  Vector Concatenate/1 -> CAN Stuffer/1(frame)
  Init/1 -> [Init]  "Init"
  [Init] -> MATLAB Function/1(Init)
  BusIdle/1 -> [BusIdle]
  [BusIdle] -> MATLAB Function1/2(BusIdle)
  Arbitration/1 -> [Arbitration]
  [Arbitration] -> MATLAB Function2/1(Arbitration)
  MATLAB Function/1(InitCmplt) -> [InitCmplt]  "InitCmplt"
  [InitCmplt] -> InitCmplt/1
  MATLAB Function1/1(SOF) -> [SOF]
  [SOF] -> SOF/1
  MATLAB Function2/1(ArbCmplt) -> [ArbCmplt]
  [ArbCmplt] -> "ArbCmplt "/1
  [Win] -> Win/1
  MATLAB Function2/2(Win) -> [Win]

== system CAN_Model_v8/CanNode_Receiver/CanNode/Frame Formatter/Control Bits ==
  Control Bits : Concatenate  NumInputs=3
  DLC : Constant  Value=[1,0,0,0]
  IDE : Constant  Value=0
  Reserved : Constant  Value=0
  ControlBits : Outport
  wires:
  DLC/1 -> Control Bits/3
  IDE/1 -> Control Bits/1
  Reserved/1 -> Control Bits/2
  Control Bits/1 -> ControlBits/1

== system CAN_Model_v8/CanNode_Receiver/CanNode/Frame Formatter/FrameStuffer ==
  FrameToStuff : Inport
  RestOfTheFrame : Inport  Port=2
  CAN Stuffer : MATLAB Function  TreatAsAtomicUnit=on
  MATLAB Function : MATLAB Function  TreatAsAtomicUnit=on
  Scope : Scope
  Scope1 : Scope
  VectorLength : MATLAB Function  TreatAsAtomicUnit=on
  VectorLength1 : MATLAB Function  TreatAsAtomicUnit=on
  TxFrame : Outport
  TxFrame_Length : Outport  Port=2
  wires:
  MATLAB Function/2(LEN_C) -> TxFrame_Length/1
  MATLAB Function/1(C) -> TxFrame/1
  RestOfTheFrame/1 -> VectorLength/1(Vector), MATLAB Function/3(B)
  VectorLength/1(Length) -> MATLAB Function/4(LEN_B)
  FrameToStuff/1 -> VectorLength1/1(Vector), CAN Stuffer/1(frame)
  CAN Stuffer/1(stuffed_frame) -> MATLAB Function/1(A)
  CAN Stuffer/2(stuffed_frame_length) -> Scope/1, MATLAB Function/2(LEN_A)
  VectorLength1/1(Length) -> Scope1/1

== system CAN_Model_v8/CanNode_Sender/CanNode/Frame Formatter/Control Bits ==
  Control Bits : Concatenate  NumInputs=3
  DLC : Constant  Value=[1,0,0,0]
  IDE : Constant  Value=0
  Reserved : Constant  Value=0
  ControlBits : Outport
  wires:
  DLC/1 -> Control Bits/3
  IDE/1 -> Control Bits/1
  Reserved/1 -> Control Bits/2
  Control Bits/1 -> ControlBits/1

== system CAN_Model_v8/CanNode_Sender/CanNode/Frame Formatter/FrameStuffer ==
  FrameToStuff : Inport
  RestOfTheFrame : Inport  Port=2
  CAN Stuffer : MATLAB Function  TreatAsAtomicUnit=on
  MATLAB Function : MATLAB Function  TreatAsAtomicUnit=on
  Scope : Scope
  Scope1 : Scope
  VectorLength : MATLAB Function  TreatAsAtomicUnit=on
  VectorLength1 : MATLAB Function  TreatAsAtomicUnit=on
  TxFrame : Outport
  TxFrame_Length : Outport  Port=2
  wires:
  MATLAB Function/2(LEN_C) -> TxFrame_Length/1
  MATLAB Function/1(C) -> TxFrame/1
  RestOfTheFrame/1 -> VectorLength/1(Vector), MATLAB Function/3(B)
  VectorLength/1(Length) -> MATLAB Function/4(LEN_B)
  FrameToStuff/1 -> VectorLength1/1(Vector), CAN Stuffer/1(frame)
  CAN Stuffer/1(stuffed_frame) -> MATLAB Function/1(A)
  CAN Stuffer/2(stuffed_frame_length) -> Scope/1, MATLAB Function/2(LEN_A)
  VectorLength1/1(Length) -> Scope1/1

== system CAN_Model_v8/CanTrafficSimulator/CanNode/Frame Formatter/Control Bits ==
  Control Bits : Concatenate  NumInputs=3
  DLC : Constant  Value=[1,0,0,0]
  IDE : Constant  Value=0
  Reserved : Constant  Value=0
  ControlBits : Outport
  wires:
  DLC/1 -> Control Bits/3
  IDE/1 -> Control Bits/1
  Reserved/1 -> Control Bits/2
  Control Bits/1 -> ControlBits/1

== system CAN_Model_v8/CanTrafficSimulator/CanNode/Frame Formatter/FrameStuffer ==
  FrameToStuff : Inport
  RestOfTheFrame : Inport  Port=2
  CAN Stuffer : MATLAB Function  TreatAsAtomicUnit=on
  MATLAB Function : MATLAB Function  TreatAsAtomicUnit=on
  Scope : Scope
  Scope1 : Scope
  VectorLength : MATLAB Function  TreatAsAtomicUnit=on
  VectorLength1 : MATLAB Function  TreatAsAtomicUnit=on
  TxFrame : Outport
  TxFrame_Length : Outport  Port=2
  wires:
  MATLAB Function/2(LEN_C) -> TxFrame_Length/1
  MATLAB Function/1(C) -> TxFrame/1
  RestOfTheFrame/1 -> VectorLength/1(Vector), MATLAB Function/3(B)
  VectorLength/1(Length) -> MATLAB Function/4(LEN_B)
  FrameToStuff/1 -> VectorLength1/1(Vector), CAN Stuffer/1(frame)
  CAN Stuffer/1(stuffed_frame) -> MATLAB Function/1(A)
  CAN Stuffer/2(stuffed_frame_length) -> Scope/1, MATLAB Function/2(LEN_A)
  VectorLength1/1(Length) -> Scope1/1

== matlab function CAN_Model_v8/CanNode_Sender/CanNode/Triggered Subsystem1/MATLAB Function ==
  data: Init input; InitCmplt output; Bus input; index input; next_index output
function [InitCmplt, next_index] = BusIdleSensing(Init, Bus, index)

InitCmplt = 0;

if Init == 1
    if Bus == 1
        if index < 10 %Number of one to wait for EOF (after 11 ones)
            next_index = index + 1;
        else
            next_index = 0;
            InitCmplt = 1;
        end
    else
        next_index = 0;
    end
else
   next_index = 0;
end

end

== matlab function CAN_Model_v8/CanNode_Sender/CanNode/Transmitter/CAN_Transmission ==
  data: frame input; frame_length input; enable input; serial output; tx_completed output; index input; next_index output
function [serial,  tx_completed ,next_index]  = fcn(frame, frame_length, enable, index)

if enable == 1
    if index > frame_length
        serial = 1;
        tx_completed = 1;
        next_index = 1;
    else
        serial = frame(index);
        next_index = index + 1;
        tx_completed = 0;
    end
else
    tx_completed = 0;
    serial = 1;
    next_index = 1;
end

end

== stateflow chart CAN_Model_v8/CanNode_Sender/CanNode/Chart ==
  settings: sampleTime=0.2  executeAtInitialization=1
  state Init
  state Rx
  state BusIdle
  state Arbitration
  state Tx
  Init -> Init [order 2] : [InitCmplt == 0]
  (default) -> Init
  Init -> BusIdle [order 1] : [InitCmplt == 1]
  Rx -> Rx [order 2] : [EOF == 0]
  BusIdle -> Rx [order 2] : [ReadyToSend == 0 && SOF == 1]
  Rx -> BusIdle [order 1] : [EOF == 1]
  BusIdle -> BusIdle [order 3] : [ReadyToSend == 0 && SOF == 0]
  Arbitration -> Rx [order 1] : [ArbCmplt ==1 && Win == 0]
  Tx -> BusIdle [order 2] : [EOF == 1]
  BusIdle -> Arbitration [order 1] : [ReadyToSend > 0]
  Arbitration -> Tx [order 2] : [ArbCmplt ==1 && Win == 1]
  Arbitration -> Arbitration [order 3] : [ArbCmplt == 0]
  Tx -> Tx [order 1] : [EOF == 0]
  data: Init output boolean; BusIdle output boolean; Arbitration output boolean; Tx output boolean; Rx output boolean; ReadyToSend input; InitCmplt input; SOF input; ArbCmplt input; Win input; EOF input
  events: Start input FALLING_EDGE_EVENT

== matlab function CAN_Model_v8/CanNode_Sender/CanNode/Triggered Subsystem1/MATLAB Function1 ==
  data: Bus input; SOF output; BusIdle input
function SOF = SOF_Detection(Bus, BusIdle)

if BusIdle == 1 %Checks the current state of the FSM
    if Bus == 0
        SOF = 1; %SOF Detected, the flag goes to One!
    else
        SOF = 0;    
    end
else
    SOF = 0;
end

end

== matlab function CAN_Model_v8/CanNode_Sender/CanNode/Triggered Subsystem1/MATLAB Function2 ==
  data: ArbCmplt output; Win output; Arbitration input; Bus input; ID input; ID_Lenght input; next_index output; index input
function [ArbCmplt, Win, next_index] = arbitration(Arbitration, Bus, ID, ID_Lenght, index)

ArbCmplt = 0;
Win = 0;
next_index = 1;

if Arbitration == 1
    if index <= ID_Lenght
        if ID(index) == Bus
            next_index = index + 1;
        else
            Win = 0;
            ArbCmplt = 1;
        end
    else
        next_index = 1;
        Win = 1;
        ArbCmplt = 1;
    end    
    
else next_index = 1;
    
end
end

== matlab function CAN_Model_v8/CanNode_Sender/CanNode/Triggered Subsystem1/CAN Stuffer ==
  data: frame input; stuffed_frame output; stuffed_frame_length output
function [stuffed_frame, stuffed_frame_length] = CANstuffer(frame)

NumOfZeros = 0;
NumOfOnes = 0;
NumOfStuffedBits = 0;

stuffed_frame = zeros(135,1);

for i = 1 : length(frame)
    if frame(i) == 0
        NumOfZeros = NumOfZeros + 1;
        NumOfOnes = 0;
    else
        NumOfOnes = NumOfOnes + 1;
        NumOfZeros = 0;
    end
    
    if NumOfZeros == 5
        NumOfZeros = 0;
        NumOfOnes = NumOfOnes + 1;
        
        %Appending the stuffed ONE
        stuffed_frame(i + NumOfStuffedBits) = frame(i);
        NumOfStuffedBits = NumOfStuffedBits + 1;
        stuffed_frame(i + NumOfStuffedBits) = 1;
        
    elseif NumOfOnes == 5
        NumOfOnes = 0;
        NumOfZeros = NumOfZeros + 1;
        
        %Appending the stuffed ZERO
        stuffed_frame(i + NumOfStuffedBits) = frame(i);
        NumOfStuffedBits = NumOfStuffedBits + 1;
        stuffed_frame(i + NumOfStuffedBits) = 0;
        
    else
        stuffed_frame(i + NumOfStuffedBits) = frame(i); 
    end
end
stuffed_frame_length = length(frame) + NumOfStuffedBits;
end

== stateflow chart CAN_Model_v8/CanTrafficSimulator/CanNode/Chart ==
  settings: sampleTime=0.2  executeAtInitialization=1
  state Init
  state Rx
  state BusIdle
  state Arbitration
  state Tx
  Init -> Init [order 2] : [InitCmplt == 0]
  (default) -> Init
  Init -> BusIdle [order 1] : [InitCmplt == 1]
  Rx -> Rx [order 2] : [EOF == 0]
  BusIdle -> Rx [order 2] : [ReadyToSend == 0 && SOF == 1]
  Rx -> BusIdle [order 1] : [EOF == 1]
  BusIdle -> BusIdle [order 3] : [ReadyToSend == 0 && SOF == 0]
  Arbitration -> Rx [order 1] : [ArbCmplt ==1 && Win == 0]
  Tx -> BusIdle [order 2] : [EOF == 1]
  BusIdle -> Arbitration [order 1] : [ReadyToSend > 0]
  Arbitration -> Tx [order 2] : [ArbCmplt ==1 && Win == 1]
  Arbitration -> Arbitration [order 3] : [ArbCmplt == 0]
  Tx -> Tx [order 1] : [EOF == 0]
  data: Init output boolean; BusIdle output boolean; Arbitration output boolean; Tx output boolean; Rx output boolean; ReadyToSend input; InitCmplt input; SOF input; ArbCmplt input; Win input; EOF input
  events: Start input FALLING_EDGE_EVENT

== matlab function CAN_Model_v8/CanNode_Sender/CanNode/Frame Formatter/FrameStuffer/CAN Stuffer ==
  data: stuffed_frame output; stuffed_frame_length output; frame input
function [stuffed_frame, stuffed_frame_length] = CANstuffer(frame)

NumOfZeros = 0;
NumOfOnes = 0;
NumOfStuffedBits = 0;

stuffed_frame = zeros(135,1);

for i = 1 : length(frame)
    if frame(i) == 0
        NumOfZeros = NumOfZeros + 1;
        NumOfOnes = 0;
    else
        NumOfOnes = NumOfOnes + 1;
        NumOfZeros = 0;
    end
    
    if NumOfZeros == 5
        NumOfZeros = 0;
        NumOfOnes = NumOfOnes + 1;
        
        %Appending the stuffed ONE
        stuffed_frame(i + NumOfStuffedBits) = frame(i);
        NumOfStuffedBits = NumOfStuffedBits + 1;
        stuffed_frame(i + NumOfStuffedBits) = 1;
        
    elseif NumOfOnes == 5
        NumOfOnes = 0;
        NumOfZeros = NumOfZeros + 1;
        
        %Appending the stuffed ZERO
        stuffed_frame(i + NumOfStuffedBits) = frame(i);
        NumOfStuffedBits = NumOfStuffedBits + 1;
        stuffed_frame(i + NumOfStuffedBits) = 0;
        
    else
        stuffed_frame(i + NumOfStuffedBits) = frame(i); 
    end
end
stuffed_frame_length = length(frame) + NumOfStuffedBits;
end

== matlab function CAN_Model_v8/CanNode_Sender/CanNode/Frame Formatter/FrameStuffer/MATLAB Function ==
  data: A input; C output; LEN_A input; B input; LEN_B input; LEN_C output
function [C, LEN_C] = vectorAppend(A, LEN_A, B, LEN_B)

C = zeros(135,1);

for i = 1 : LEN_A
    C(i) = A(i);
end

for i = 1 : LEN_B
    C(LEN_A + i) = B(i);
end

LEN_C = LEN_A + LEN_B;
end

== matlab function CAN_Model_v8/CanNode_Sender/CanNode/Frame Formatter/FrameStuffer/VectorLength ==
  data: Vector input; Length output
function Length = VectorLength(Vector)
Length = length(Vector);
end

== matlab function CAN_Model_v8/CanNode_Sender/CanNode/Frame Formatter/FrameStuffer/VectorLength1 ==
  data: Vector input; Length output
function Length = VectorLength(Vector)
Length = length(Vector);
end

== matlab function CAN_Model_v8/CanTrafficSimulator/CanNode/Frame Formatter/FrameStuffer/CAN Stuffer ==
  data: stuffed_frame output; stuffed_frame_length output; frame input
function [stuffed_frame, stuffed_frame_length] = CANstuffer(frame)

NumOfZeros = 0;
NumOfOnes = 0;
NumOfStuffedBits = 0;

stuffed_frame = zeros(135,1);

for i = 1 : length(frame)
    if frame(i) == 0
        NumOfZeros = NumOfZeros + 1;
        NumOfOnes = 0;
    else
        NumOfOnes = NumOfOnes + 1;
        NumOfZeros = 0;
    end
    
    if NumOfZeros == 5
        NumOfZeros = 0;
        NumOfOnes = NumOfOnes + 1;
        
        %Appending the stuffed ONE
        stuffed_frame(i + NumOfStuffedBits) = frame(i);
        NumOfStuffedBits = NumOfStuffedBits + 1;
        stuffed_frame(i + NumOfStuffedBits) = 1;
        
    elseif NumOfOnes == 5
        NumOfOnes = 0;
        NumOfZeros = NumOfZeros + 1;
        
        %Appending the stuffed ZERO
        stuffed_frame(i + NumOfStuffedBits) = frame(i);
        NumOfStuffedBits = NumOfStuffedBits + 1;
        stuffed_frame(i + NumOfStuffedBits) = 0;
        
    else
        stuffed_frame(i + NumOfStuffedBits) = frame(i); 
    end
end
stuffed_frame_length = length(frame) + NumOfStuffedBits;
end

== matlab function CAN_Model_v8/CanTrafficSimulator/CanNode/Frame Formatter/FrameStuffer/MATLAB Function ==
  data: A input; C output; LEN_A input; B input; LEN_B input; LEN_C output
function [C, LEN_C] = vectorAppend(A, LEN_A, B, LEN_B)

C = zeros(135,1);

for i = 1 : LEN_A
    C(i) = A(i);
end

for i = 1 : LEN_B
    C(LEN_A + i) = B(i);
end

LEN_C = LEN_A + LEN_B;
end

== matlab function CAN_Model_v8/CanTrafficSimulator/CanNode/Frame Formatter/FrameStuffer/VectorLength ==
  data: Vector input; Length output
function Length = VectorLength(Vector)
Length = length(Vector);
end

== matlab function CAN_Model_v8/CanTrafficSimulator/CanNode/Frame Formatter/FrameStuffer/VectorLength1 ==
  data: Vector input; Length output
function Length = VectorLength(Vector)
Length = length(Vector);
end

== matlab function CAN_Model_v8/CanTrafficSimulator/CanNode/Receiver/MATLAB BusRxAndDestuff ==
  data: Bus input; EOF output; ACK output; Enable input; AckEnable input; Frame input; Index input; Error output; DeStuffedFrame output; NextFrame output; NextIndex output; Count input; NextCount output; Jump input; NextJump output
function [EOF, ACK, Error, DeStuffedFrame, NextFrame, NextIndex, NextCount, NextJump] = BusRxAndDestuff(Bus, Enable, AckEnable, Frame, Index, Count, Jump)

DeStuffedFrame = zeros(111,1);
NextCount = 0;
NextFrame = zeros(111,1);
EOF = 0;
Error = 0;
NextIndex = 2;
NextJump = 0;
ACK = 1;

if Enable == 1
    if Index <= 111
        NextFrame = Frame;
        if (Index <= 98) || (Count == 4)
            if (Index == 1) || (Jump == 1)
                NextFrame(Index) = Bus;
                NextIndex = Index + 1;
            else
                if Count == 4
                    NextIndex = Index;
                    NextCount = 0;
                    NextJump = 1;
                else
                    NextFrame(Index) = Bus;
                    NextIndex = Index + 1;
                    if Bus == NextFrame(Index - 1)
                        NextCount = Count + 1;
                    else
                        NextCount = 0;
                    end
                end
            end
        else
            if(Index == 99) && (AckEnable == 1)
                ACK = 0;
            end
            NextFrame(Index) = Bus;
            NextIndex = Index + 1;
        end
    else
        EOF = 1;
        DeStuffedFrame = Frame;
    end
end
end
